simulink library "FMT_Model_Lib"  (R2018b)
settings: Solver=VariableStepAuto  StartTime=0.0  StopTime=10.0  RelTol=1e-3
undefined symbols (not defined in the file or in its folder): DiscIntNeverNeededParam, Newton, Raphson
libraries: $bdroot x14
(part 2 of 2)

== system FMT_Model_Lib/Quaternion/DCM To Quaternion/Negative Trace/Maximum Value at DCM(1,1) ==
  DCM : Inport
  Action Port : ActionPort  PropagateVarSize=During execution  ActionType=else
  Demux : Demux  Outputs=3
  Gain : Gain  Gain=0.5  SaturateOnIntegerOverflow=on  OutDataTypeStr=Inherit: Same as input  ParamDataTypeStr=Inherit: Same as input
  Gain1 : Gain  SaturateOnIntegerOverflow=on  OutDataTypeStr=Inherit: Same as input  ParamDataTypeStr=Inherit: Same as input
  Gain2 : Gain  SaturateOnIntegerOverflow=on  OutDataTypeStr=Inherit: Same as input  ParamDataTypeStr=Inherit: Same as input
  Gain3 : Gain  SaturateOnIntegerOverflow=on  OutDataTypeStr=Inherit: Same as input  ParamDataTypeStr=Inherit: Same as input
  Mux : Mux
  Mux1 : Mux  Inputs=3
  Product : Product  SaturateOnIntegerOverflow=on  InputSameDT=on  OutDataTypeStr=Inherit: Same as first input
  cos(phi)sin(theta)cos(psi) + sin(phi)sin(psi) -sin(theta) : Subsystem
  cos(theta)sin(phi) - (cos(phi)sin(theta)sin(psi) - sin(phi)cos(psi)) : Subsystem
  cos(theta)sin(psi) + (sin(phi)sin(theta)cos(psi) - cos(phi)sin(psi)) : Subsystem
  if s~=0; s=0.5/s : Subsystem
  sqrt : Sqrt  AlgorithmType=Newton-Raphson  SaturateOnIntegerOverflow=on
  u(1) -(u(5)+u(9)) +1 : Subsystem
  qw qx qy qz : Outport
  wires:
  DCM/1 -> u(1) -(u(5)+u(9)) +1/1(DCM), cos(theta)sin(psi) + (sin(phi)sin(theta)cos(psi) - cos(phi)sin(psi))/1(DCM), cos(theta)sin(phi) - (cos(phi)sin(theta)sin(psi) - sin(phi)cos(psi))/1(DCM), cos(phi)sin(theta)cos(psi) + sin(phi)sin(psi) -sin(theta)/1(DCM)
  cos(theta)sin(psi) + (sin(phi)sin(theta)cos(psi) - cos(phi)sin(psi))/1(u(4)+u(2)) -> Mux1/1
  cos(phi)sin(theta)cos(psi) + sin(phi)sin(psi) -sin(theta)/1(u(3)+u(7)) -> Mux1/2
  cos(theta)sin(phi) - (cos(phi)sin(theta)sin(psi) - sin(phi)cos(psi))/1(u(8)-u(6)) -> Mux1/3
  Mux/1 -> qw qx qy qz/1
  u(1) -(u(5)+u(9)) +1/1(out) -> sqrt/1
  sqrt/1 -> Gain/1, if s~=0; s=0.5/s/1(s)
  Mux1/1 -> Product/2
  Demux/1 -> Gain1/1
  Demux/3 -> Gain3/1
  Demux/2 -> Gain2/1
  Gain1/1 -> Mux/3
  Gain2/1 -> Mux/4
  Gain3/1 -> Mux/1
  Product/1 -> Demux/1
  Gain/1 -> Mux/2
  if s~=0; s=0.5/s/1("s ") -> Product/1

== system FMT_Model_Lib/Quaternion/DCM To Quaternion/Negative Trace/Maximum Value at DCM(2,2) ==
  DCM : Inport
  Action Port : ActionPort  PropagateVarSize=During execution  ActionType=then
  Demux : Demux  Outputs=3
  Gain : Gain  Gain=0.5  SaturateOnIntegerOverflow=on  OutDataTypeStr=Inherit: Same as input  ParamDataTypeStr=Inherit: Same as input
  Gain1 : Gain  SaturateOnIntegerOverflow=on  OutDataTypeStr=Inherit: Same as input  ParamDataTypeStr=Inherit: Same as input
  Gain3 : Gain  SaturateOnIntegerOverflow=on  OutDataTypeStr=Inherit: Same as input  ParamDataTypeStr=Inherit: Same as input
  Gain4 : Gain  SaturateOnIntegerOverflow=on  OutDataTypeStr=Inherit: Same as input  ParamDataTypeStr=Inherit: Same as input
  Mux : Mux
  Mux1 : Mux  Inputs=3
  Product : Product  SaturateOnIntegerOverflow=on  InputSameDT=on  OutDataTypeStr=Inherit: Same as first input
  cos(phi)sin(theta)cos(psi) + sin(phi)sin(psi) +sin(theta) : Subsystem
  cos(theta)sin(phi) + (cos(phi)sin(theta)sin(psi) - sin(phi)cos(psi)) : Subsystem
  cos(theta)sin(psi) + (sin(phi)sin(theta)cos(psi) - cos(phi)sin(psi)) : Subsystem
  if s~=0; s=0.5/s : Subsystem
  sqrt : Sqrt  AlgorithmType=Newton-Raphson  SaturateOnIntegerOverflow=on
  u(5) -(u(1)+u(9)) +1 : Subsystem
  qw qx qy qz : Outport
  wires:
  Mux1/1 -> Product/1
  DCM/1 -> u(5) -(u(1)+u(9)) +1/1(DCM), cos(phi)sin(theta)cos(psi) + sin(phi)sin(psi) +sin(theta)/1(DCM), cos(theta)sin(psi) + (sin(phi)sin(theta)cos(psi) - cos(phi)sin(psi))/1(DCM), cos(theta)sin(phi) + (cos(phi)sin(theta)sin(psi) - sin(phi)cos(psi))/1(DCM)
  cos(theta)sin(psi) + (sin(phi)sin(theta)cos(psi) - cos(phi)sin(psi))/1(u(4)+u(2)) -> Mux1/1
  cos(theta)sin(phi) + (cos(phi)sin(theta)sin(psi) - sin(phi)cos(psi))/1(u(8)+u(6)) -> Mux1/2
  cos(phi)sin(theta)cos(psi) + sin(phi)sin(psi) +sin(theta)/1(u(3)-u(7)) -> Mux1/3
  Mux/1 -> qw qx qy qz/1
  u(5) -(u(1)+u(9)) +1/1(out) -> sqrt/1
  Gain/1 -> Mux/3
  Product/1 -> Demux/1
  Demux/1 -> Gain1/1
  Demux/2 -> Gain3/1
  Demux/3 -> Gain4/1
  Gain1/1 -> Mux/2
  Gain3/1 -> Mux/4
  Gain4/1 -> Mux/1
  if s~=0; s=0.5/s/1("s ") -> Product/2
  sqrt/1 -> if s~=0; s=0.5/s/1(s), Gain/1

== system FMT_Model_Lib/Quaternion/DCM To Quaternion/Negative Trace/Maximum Value at DCM(3,3) ==
  DCM : Inport
  Action Port : ActionPort  PropagateVarSize=During execution  ActionType=elseif
  Demux : Demux  Outputs=3
  Gain : Gain  Gain=0.5  SaturateOnIntegerOverflow=on  OutDataTypeStr=Inherit: Same as input  ParamDataTypeStr=Inherit: Same as input
  Gain1 : Gain  SaturateOnIntegerOverflow=on  OutDataTypeStr=Inherit: Same as input  ParamDataTypeStr=Inherit: Same as input
  Gain2 : Gain  SaturateOnIntegerOverflow=on  OutDataTypeStr=Inherit: Same as input  ParamDataTypeStr=Inherit: Same as input
  Gain3 : Gain  SaturateOnIntegerOverflow=on  OutDataTypeStr=Inherit: Same as input  ParamDataTypeStr=Inherit: Same as input
  Mux : Mux
  Mux1 : Mux  Inputs=3
  Product : Product  SaturateOnIntegerOverflow=on  InputSameDT=on  OutDataTypeStr=Inherit: Same as first input
  cos(phi)sin(theta)cos(psi) + sin(phi)sin(psi) -sin(theta) : Subsystem
  cos(theta)sin(phi) + (cos(phi)sin(theta)sin(psi) - sin(phi)cos(psi)) : Subsystem
  cos(theta)sin(psi) - (sin(phi)sin(theta)cos(psi) - cos(phi)sin(psi)) : Subsystem
  if s~=0; s=0.5/s : Subsystem
  sqrt : Sqrt  AlgorithmType=Newton-Raphson  SaturateOnIntegerOverflow=on
  u(9) -(u(1)+u(5)) +1 : Subsystem
  qw qx qy qz : Outport
  wires:
  Mux1/1 -> Product/1
  DCM/1 -> u(9) -(u(1)+u(5)) +1/1(DCM), cos(theta)sin(psi) - (sin(phi)sin(theta)cos(psi) - cos(phi)sin(psi))/1(DCM), cos(theta)sin(phi) + (cos(phi)sin(theta)sin(psi) - sin(phi)cos(psi))/1(DCM), cos(phi)sin(theta)cos(psi) + sin(phi)sin(psi) -sin(theta)/1(DCM)
  cos(phi)sin(theta)cos(psi) + sin(phi)sin(psi) -sin(theta)/1(u(3)+u(7)) -> Mux1/1
  cos(theta)sin(phi) + (cos(phi)sin(theta)sin(psi) - sin(phi)cos(psi))/1(u(8)+u(6)) -> Mux1/2
  cos(theta)sin(psi) - (sin(phi)sin(theta)cos(psi) - cos(phi)sin(psi))/1(u(4)-u(2)) -> Mux1/3
  Mux/1 -> qw qx qy qz/1
  u(9) -(u(1)+u(5)) +1/1(out) -> sqrt/1
  sqrt/1 -> Gain/1, if s~=0; s=0.5/s/1(s)
  Product/1 -> Demux/1
  Demux/1 -> Gain1/1
  Demux/3 -> Gain3/1
  Demux/2 -> Gain2/1
  Gain/1 -> Mux/4
  Gain1/1 -> Mux/2
  Gain2/1 -> Mux/3
  Gain3/1 -> Mux/1
  if s~=0; s=0.5/s/1("s ") -> Product/2

== system FMT_Model_Lib/Quaternion/DCM To Quaternion/Negative Trace/diag(DCM) ==
  DCM : Inport
  Demux : Demux  Outputs=3
  Selector : Selector  InputPortWidth=9  IndexOptions=Index vector (dialog)  Indices=[1 5 9]  OutputSizes=1
  u(1) : Outport
  u(5) : Outport  Port=2
  u(9) : Outport  Port=3
  wires:
  DCM/1 -> Selector/1
  Demux/1 -> u(1)/1
  Demux/2 -> u(5)/1
  Demux/3 -> u(9)/1
  Selector/1 -> Demux/1

== system FMT_Model_Lib/Quaternion/DCM To Quaternion/Positive Trace/cos(phi)sin(theta)cos(psi) + sin(phi)sin(psi) +sin(theta) ==
  DCM : Inport
  Add : Sum  Inputs=+-|
  Demux : Demux  Outputs=2
  Selector : Selector  InputPortWidth=9  IndexOptions=Index vector (dialog)  Indices=[3 7]  OutputSizes=1
  u(3)-u(7) : Outport
  wires:
  DCM/1 -> Selector/1
  Add/1 -> u(3)-u(7)/1
  Selector/1 -> Demux/1
  Demux/2 -> Add/2
  Demux/1 -> Add/1

== system FMT_Model_Lib/Quaternion/DCM To Quaternion/Positive Trace/cos(theta)sin(phi) - (cos(phi)sin(theta)sin(psi) - sin(phi)cos(psi)) ==
  DCM : Inport
  Add : Sum  Inputs=|-+
  Demux : Demux  Outputs=2
  Selector : Selector  InputPortWidth=9  IndexOptions=Index vector (dialog)  Indices=[6 8]  OutputSizes=1
  u(8)-u(6) : Outport
  wires:
  Add/1 -> u(8)-u(6)/1
  DCM/1 -> Selector/1
  Demux/1 -> Add/1
  Demux/2 -> Add/2
  Selector/1 -> Demux/1

== system FMT_Model_Lib/Quaternion/DCM To Quaternion/Positive Trace/cos(theta)sin(psi) - (sin(phi)sin(theta)cos(psi) - cos(phi)sin(psi)) ==
  DCM : Inport
  Add : Sum  Inputs=|-+
  Demux : Demux  Outputs=2
  Selector : Selector  InputPortWidth=9  IndexOptions=Index vector (dialog)  Indices=[2 4]  OutputSizes=1
  u(4)-u(2) : Outport
  wires:
  Add/1 -> u(4)-u(2)/1
  DCM/1 -> Selector/1
  Selector/1 -> Demux/1
  Demux/1 -> Add/1
  Demux/2 -> Add/2

== system FMT_Model_Lib/Quaternion/DCM To Quaternion/Negative Trace/Maximum Value at DCM(1,1)/cos(phi)sin(theta)cos(psi) + sin(phi)sin(psi) -sin(theta) ==
  DCM : Inport
  Add : Sum  Inputs=++|
  Demux : Demux  Outputs=2
  Selector : Selector  InputPortWidth=9  IndexOptions=Index vector (dialog)  Indices=[3 7]  OutputSizes=1
  u(3)+u(7) : Outport
  wires:
  DCM/1 -> Selector/1
  Add/1 -> u(3)+u(7)/1
  Demux/2 -> Add/2
  Demux/1 -> Add/1
  Selector/1 -> Demux/1

== system FMT_Model_Lib/Quaternion/DCM To Quaternion/Negative Trace/Maximum Value at DCM(1,1)/cos(theta)sin(phi) - (cos(phi)sin(theta)sin(psi) - sin(phi)cos(psi)) ==
  DCM : Inport
  Add : Sum  Inputs=|-+
  Demux : Demux  Outputs=2
  Selector : Selector  InputPortWidth=9  IndexOptions=Index vector (dialog)  Indices=[6 8]  OutputSizes=1
  u(8)-u(6) : Outport
  wires:
  DCM/1 -> Selector/1
  Add/1 -> u(8)-u(6)/1
  Selector/1 -> Demux/1
  Demux/1 -> Add/1
  Demux/2 -> Add/2

== system FMT_Model_Lib/Quaternion/DCM To Quaternion/Negative Trace/Maximum Value at DCM(1,1)/cos(theta)sin(psi) + (sin(phi)sin(theta)cos(psi) - cos(phi)sin(psi)) ==
  DCM : Inport
  Add : Sum  Inputs=|++
  Demux : Demux  Outputs=2
  Selector : Selector  InputPortWidth=9  IndexOptions=Index vector (dialog)  Indices=[2 4]  OutputSizes=1
  u(4)+u(2) : Outport
  wires:
  Add/1 -> u(4)+u(2)/1
  DCM/1 -> Selector/1
  Selector/1 -> Demux/1
  Demux/1 -> Add/1
  Demux/2 -> Add/2

== system FMT_Model_Lib/Quaternion/DCM To Quaternion/Negative Trace/Maximum Value at DCM(1,1)/if s~=0; s=0.5//s ==
  s : Inport
  Constant1 : Constant  Value=0.5  OutDataTypeStr=Inherit: Inherit via back propagation
  Constant2 : Constant  Value=[0 1]  OutDataTypeStr=Inherit: Inherit via back propagation
  Demux : Demux  Outputs=2
  Mux : Mux  Inputs=2
  Product : Product  Inputs=*/  RndMeth=Zero
  Switch : Switch  Criteria=u2 ~= 0  SaturateOnIntegerOverflow=on  InputSameDT=on
  "s " : Outport
  wires:
  Demux/1 -> Product/1
  Demux/2 -> Product/2
  Constant1/1 -> Mux/1
  Mux/1 -> Switch/1
  s/1 -> Switch/2, Mux/2
  Switch/1 -> Demux/1
  Constant2/1 -> Switch/3
  Product/1 -> "s "/1

== system FMT_Model_Lib/Quaternion/DCM To Quaternion/Negative Trace/Maximum Value at DCM(1,1)/u(1) -(u(5)+u(9)) +1 ==
  DCM : Inport
  Add : Sum  Inputs=+--+
  Constant : Constant  OutDataTypeStr=Inherit: Inherit via back propagation
  Demux : Demux  Outputs=3
  Selector : Selector  InputPortWidth=9  IndexOptions=Index vector (dialog)  Indices=[1 5 9]  OutputSizes=1
  out : Outport
  wires:
  Add/1 -> out/1
  DCM/1 -> Selector/1
  Constant/1 -> Add/4
  Selector/1 -> Demux/1
  Demux/2 -> Add/2
  Demux/1 -> Add/1
  Demux/3 -> Add/3

== system FMT_Model_Lib/Quaternion/DCM To Quaternion/Negative Trace/Maximum Value at DCM(2,2)/cos(phi)sin(theta)cos(psi) + sin(phi)sin(psi) +sin(theta) ==
  DCM : Inport
  Add : Sum  Inputs=+-|
  Demux : Demux  Outputs=2
  Selector : Selector  InputPortWidth=9  IndexOptions=Index vector (dialog)  Indices=[3 7]  OutputSizes=1
  u(3)-u(7) : Outport
  wires:
  Add/1 -> u(3)-u(7)/1
  Demux/2 -> Add/2
  DCM/1 -> Selector/1
  Demux/1 -> Add/1
  Selector/1 -> Demux/1

== system FMT_Model_Lib/Quaternion/DCM To Quaternion/Negative Trace/Maximum Value at DCM(2,2)/cos(theta)sin(phi) + (cos(phi)sin(theta)sin(psi) - sin(phi)cos(psi)) ==
  DCM : Inport
  Add : Sum  Inputs=|++
  Demux : Demux  Outputs=2
  Selector : Selector  InputPortWidth=9  IndexOptions=Index vector (dialog)  Indices=[6 8]  OutputSizes=1
  u(8)+u(6) : Outport
  wires:
  Add/1 -> u(8)+u(6)/1
  DCM/1 -> Selector/1
  Selector/1 -> Demux/1
  Demux/1 -> Add/1
  Demux/2 -> Add/2

== system FMT_Model_Lib/Quaternion/DCM To Quaternion/Negative Trace/Maximum Value at DCM(2,2)/cos(theta)sin(psi) + (sin(phi)sin(theta)cos(psi) - cos(phi)sin(psi)) ==
  DCM : Inport
  Add : Sum  Inputs=|++
  Demux : Demux  Outputs=2
  Selector : Selector  InputPortWidth=9  IndexOptions=Index vector (dialog)  Indices=[2 4]  OutputSizes=1
  u(4)+u(2) : Outport
  wires:
  DCM/1 -> Selector/1
  Add/1 -> u(4)+u(2)/1
  Selector/1 -> Demux/1
  Demux/1 -> Add/1
  Demux/2 -> Add/2

== system FMT_Model_Lib/Quaternion/DCM To Quaternion/Negative Trace/Maximum Value at DCM(2,2)/if s~=0; s=0.5//s ==
  s : Inport
  Constant1 : Constant  Value=0.5  OutDataTypeStr=Inherit: Inherit via back propagation
  Constant2 : Constant  Value=[0 1]  OutDataTypeStr=Inherit: Inherit via back propagation
  Demux : Demux  Outputs=2
  Mux : Mux  Inputs=2
  Product : Product  Inputs=*/  RndMeth=Zero
  Switch : Switch  Criteria=u2 ~= 0  SaturateOnIntegerOverflow=on  InputSameDT=on
  "s " : Outport
  wires:
  Product/1 -> "s "/1
  Constant2/1 -> Switch/3
  Switch/1 -> Demux/1
  s/1 -> Mux/2, Switch/2
  Mux/1 -> Switch/1
  Constant1/1 -> Mux/1
  Demux/2 -> Product/2
  Demux/1 -> Product/1

== system FMT_Model_Lib/Quaternion/DCM To Quaternion/Negative Trace/Maximum Value at DCM(2,2)/u(5) -(u(1)+u(9)) +1 ==
  DCM : Inport
  Add : Sum  Inputs=-+-+
  Constant : Constant  OutDataTypeStr=Inherit: Inherit via back propagation
  Demux : Demux  Outputs=3
  Selector : Selector  InputPortWidth=9  IndexOptions=Index vector (dialog)  Indices=[1 5 9]  OutputSizes=1
  out : Outport
  wires:
  Constant/1 -> Add/4
  DCM/1 -> Selector/1
  Add/1 -> out/1
  Selector/1 -> Demux/1
  Demux/2 -> Add/2
  Demux/1 -> Add/1
  Demux/3 -> Add/3

== system FMT_Model_Lib/Quaternion/DCM To Quaternion/Negative Trace/Maximum Value at DCM(3,3)/cos(phi)sin(theta)cos(psi) + sin(phi)sin(psi) -sin(theta) ==
  DCM : Inport
  Add : Sum  Inputs=++|
  Demux : Demux  Outputs=2
  Selector : Selector  InputPortWidth=9  IndexOptions=Index vector (dialog)  Indices=[3 7]  OutputSizes=1
  u(3)+u(7) : Outport
  wires:
  Add/1 -> u(3)+u(7)/1
  DCM/1 -> Selector/1
  Demux/2 -> Add/2
  Demux/1 -> Add/1
  Selector/1 -> Demux/1

== system FMT_Model_Lib/Quaternion/DCM To Quaternion/Negative Trace/Maximum Value at DCM(3,3)/cos(theta)sin(phi) + (cos(phi)sin(theta)sin(psi) - sin(phi)cos(psi)) ==
  DCM : Inport
  Add : Sum  Inputs=|++
  Demux : Demux  Outputs=2
  Selector : Selector  InputPortWidth=9  IndexOptions=Index vector (dialog)  Indices=[6 8]  OutputSizes=1
  u(8)+u(6) : Outport
  wires:
  DCM/1 -> Selector/1
  Add/1 -> u(8)+u(6)/1
  Selector/1 -> Demux/1
  Demux/1 -> Add/1
  Demux/2 -> Add/2

== system FMT_Model_Lib/Quaternion/DCM To Quaternion/Negative Trace/Maximum Value at DCM(3,3)/cos(theta)sin(psi) - (sin(phi)sin(theta)cos(psi) - cos(phi)sin(psi)) ==
  DCM : Inport
  Add : Sum  Inputs=|-+
  Demux : Demux  Outputs=2
  Selector : Selector  InputPortWidth=9  IndexOptions=Index vector (dialog)  Indices=[2 4]  OutputSizes=1
  u(4)-u(2) : Outport
  wires:
  DCM/1 -> Selector/1
  Add/1 -> u(4)-u(2)/1
  Selector/1 -> Demux/1
  Demux/1 -> Add/1
  Demux/2 -> Add/2

== system FMT_Model_Lib/Quaternion/DCM To Quaternion/Negative Trace/Maximum Value at DCM(3,3)/if s~=0; s=0.5//s ==
  s : Inport
  Constant1 : Constant  Value=0.5  OutDataTypeStr=Inherit: Inherit via back propagation
  Constant2 : Constant  Value=[0 1]  OutDataTypeStr=Inherit: Inherit via back propagation
  Demux : Demux  Outputs=2
  Mux : Mux  Inputs=2
  Product : Product  Inputs=*/  RndMeth=Zero
  Switch : Switch  Criteria=u2 ~= 0  SaturateOnIntegerOverflow=on  InputSameDT=on
  "s " : Outport
  wires:
  Demux/1 -> Product/1
  Demux/2 -> Product/2
  Constant1/1 -> Mux/1
  Mux/1 -> Switch/1
  s/1 -> Switch/2, Mux/2
  Switch/1 -> Demux/1
  Constant2/1 -> Switch/3
  Product/1 -> "s "/1

== system FMT_Model_Lib/Quaternion/DCM To Quaternion/Negative Trace/Maximum Value at DCM(3,3)/u(9) -(u(1)+u(5)) +1 ==
  DCM : Inport
  Add : Sum  Inputs=--++
  Constant : Constant  OutDataTypeStr=Inherit: Inherit via back propagation
  Demux : Demux  Outputs=3
  Selector : Selector  InputPortWidth=9  IndexOptions=Index vector (dialog)  Indices=[1 5 9]  OutputSizes=1
  out : Outport
  wires:
  Constant/1 -> Add/4
  DCM/1 -> Selector/1
  Add/1 -> out/1
  Selector/1 -> Demux/1
  Demux/2 -> Add/2
  Demux/1 -> Add/1
  Demux/3 -> Add/3
